simulink model "Stabpendel_With_Blocks"  (Simulink 7.1)
settings: Solver=ode45  StartTime=0.0  StopTime=4.0  RelTol=1e-3
settings Model: Creator=Meisel  LastModifiedBy=Meisel

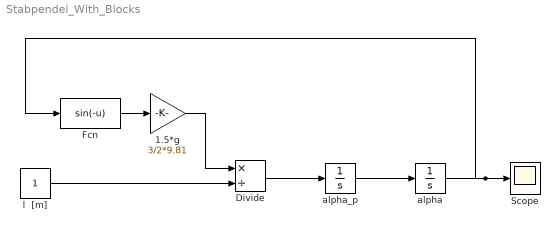
== system Stabpendel_With_Blocks ==
  1.5*g : Gain  Gain=3/2*9.81  ParameterDataType=sfix(16)  ParameterScaling=2^0  OutDataType=sfix(16)  OutScaling=2^0
  Divide : Product  Inputs=*/  OutDataType=sfix(16)  OutScaling=2^-10
  Fcn : Fcn  Expr=sin(-u)
  Scope : Scope
  alpha : Integrator  InitialCondition=30*pi/180
  alpha_p : Integrator
  l  [m] : Constant  OutDataType=sfix(16)  OutScaling=2^0
  wires:
  alpha_p/1 -> alpha/1
  alpha/1 -> Scope/1, Fcn/1
  l  [m]/1 -> Divide/2
  Divide/1 -> alpha_p/1
  Fcn/1 -> 1.5*g/1
  1.5*g/1 -> Divide/1
